simulink subsystem "MotresAJ"  (R2023b)
settings: Solver=VariableStepAuto  StartTime=0.0  StopTime=10.0  RelTol=1e-3
libraries: arduinolib x6
settings Model: Creator=Antonio  LastModifiedBy=Antonio

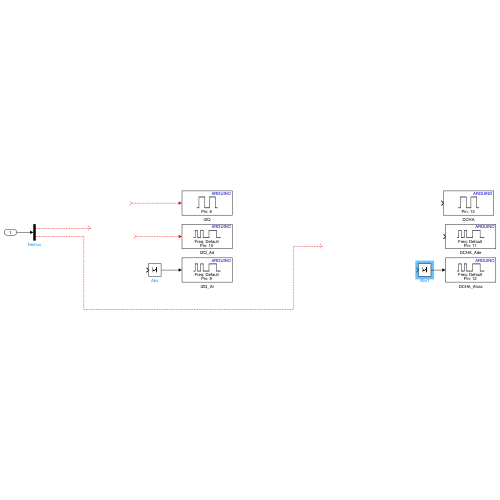
[thumbnail: Simulink's stored preview of the top-level diagram]
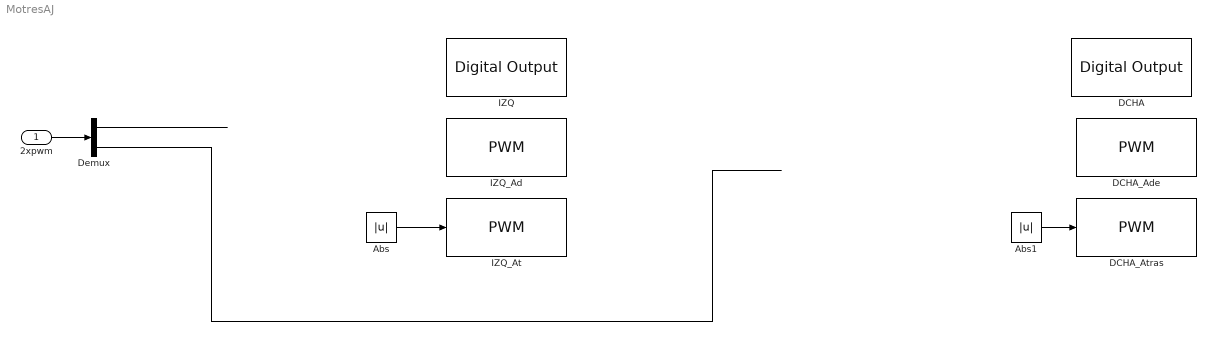
== system MotresAJ ==
  2xpwm : Inport
  Abs : Abs  SaturateOnIntegerOverflow=off
  Abs1 : Abs  SaturateOnIntegerOverflow=off
  DCHA : arduinolib/Digital Output  pinNumber=13  Direction=output  blockPlatform=arduino
  DCHA_Ade : arduinolib/PWM  pinNumber=11  frequencyType=Default  desiredFrequency=490.2  achievableFrequency=490.2
  DCHA_Atras : arduinolib/PWM  pinNumber=12  frequencyType=Default  desiredFrequency=490.2  achievableFrequency=490.2
  Demux : Demux  Outputs=2
  IZQ : arduinolib/Digital Output  pinNumber=8  Direction=output  blockPlatform=arduino
  IZQ_Ad : arduinolib/PWM  pinNumber=10  frequencyType=Default  desiredFrequency=490.2  achievableFrequency=490.2
  IZQ_At : arduinolib/PWM  pinNumber=9  frequencyType=Default  desiredFrequency=490.2  achievableFrequency=490.2
  wires:
  Abs/1 -> IZQ_At/1
  ? -> IZQ_Ad/1
  ? -> IZQ/1
  2xpwm/1 -> Demux/1
  Demux/1 -> ?
  Demux/2 -> ?
  Abs1/1 -> DCHA_Atras/1
